simulink model "Sim17"  (R2019a)
settings: Solver=FixedStepAuto  StartTime=0.0  StopTime=10.0  FixedStep=0.0001  MaxStep=0.0001  MinStep=0.0001  RelTol=1e-3
settings Model: Creator=fbleo  LastModifiedBy=fbleo
settings SolverCC: InitialStep=0.0001

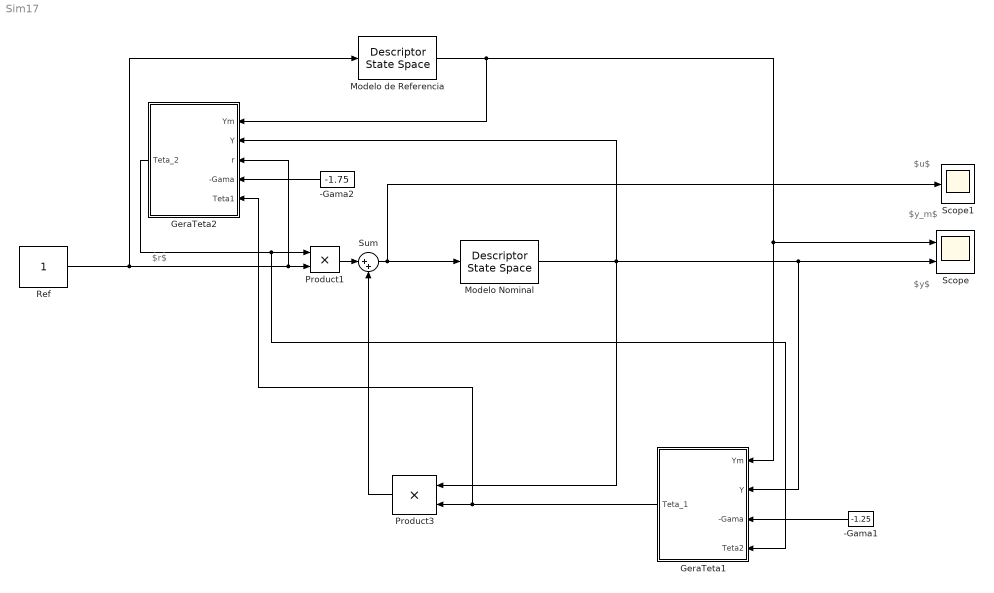
== system Sim17 ==
  note: $r$
  note: $y$
  note: $u$
  note: $y_m$
  -Gama1 : Constant  Value=-1.25
  -Gama2 : Constant  Value=-1.75
  GeraTeta1 : Subsystem
  GeraTeta2 : Subsystem
  Modelo Nominal : DescriptorStateSpace  A=-1  B=2  D=0  InitialCondition=0.5
  Modelo de Referencia : DescriptorStateSpace  A=-3  B=3  D=0  InitialCondition=0
  Product1 : Product
  Product3 : Product
  Ref : Constant
  Scope : Scope  NumInputPorts=2
  Scope1 : Scope
  Sum : Sum  Inputs=|++
  wires:
  Ref/1 -> Product1/2, GeraTeta2/3(r), Modelo de Referencia/1
  Sum/1 -> Modelo Nominal/1, Scope1/1
  GeraTeta2/1(Teta_2) -> Product1/1, GeraTeta1/4("Teta2 ")
  -Gama2/1 -> GeraTeta2/4(-Gama)
  Modelo Nominal/1 -> GeraTeta1/2(Y), Scope/2, Product3/1, GeraTeta2/2(Y)
  Product1/1 -> Sum/1
  Product3/1 -> Sum/2
  -Gama1/1 -> GeraTeta1/3(-Gama)
  Modelo de Referencia/1 -> GeraTeta1/1(Ym), Scope/1, GeraTeta2/1(Ym)
  GeraTeta1/1(Teta_1) -> GeraTeta2/5(Teta1), Product3/2

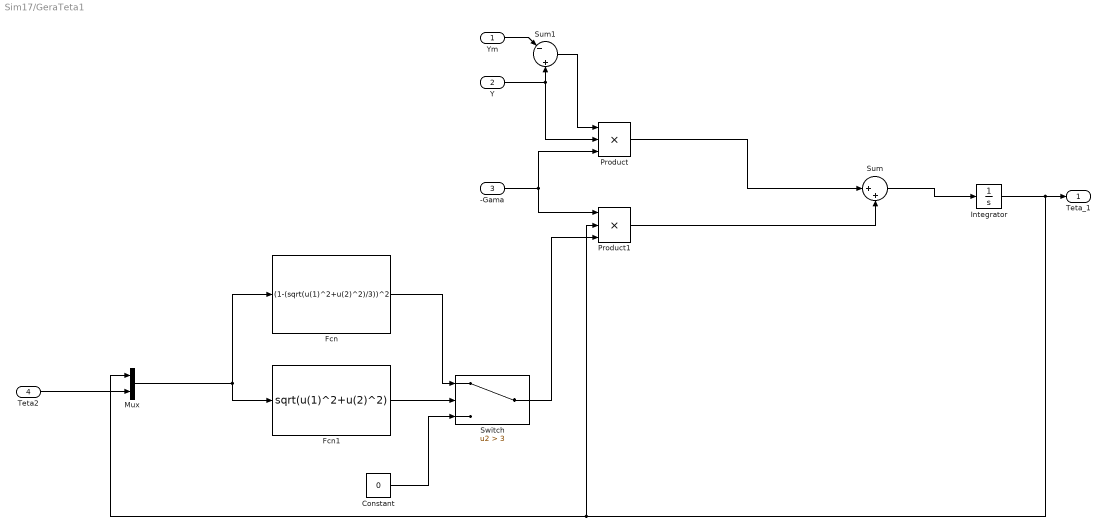
== system Sim17/GeraTeta1 ==
  Ym : Inport
  Y : Inport  Port=2
  -Gama : Inport  Port=3
  "Teta2 " : Inport  Port=4
  Constant : Constant  Value=0
  Fcn : Fcn  Expr=(1-(sqrt(u(1)^2+u(2)^2)/3))^2
  Fcn1 : Fcn  Expr=sqrt(u(1)^2+u(2)^2)
  Integrator : Integrator  InitialCondition=-0.65
  Mux : Mux  Inputs=2
  Product : Product  Inputs=3
  Product1 : Product  Inputs=3
  Sum : Sum  Inputs=|++
  Sum1 : Sum  Inputs=|-||+
  Switch : Switch  Criteria=u2 > Threshold  Threshold=3
  Teta_1 : Outport
  wires:
  Ym/1 -> Sum1/1
  Sum1/1 -> Product/1
  Y/1 -> Sum1/2, Product/2
  -Gama/1 -> Product1/1, Product/3
  Product/1 -> Sum/1
  Sum/1 -> Integrator/1
  Integrator/1 -> Mux/1, Product1/2, Teta_1/1
  "Teta2 "/1 -> Mux/2
  Switch/1 -> Product1/3
  Product1/1 -> Sum/2
  Fcn/1 -> Switch/1
  Mux/1 -> Fcn1/1, Fcn/1
  Constant/1 -> Switch/3
  Fcn1/1 -> Switch/2

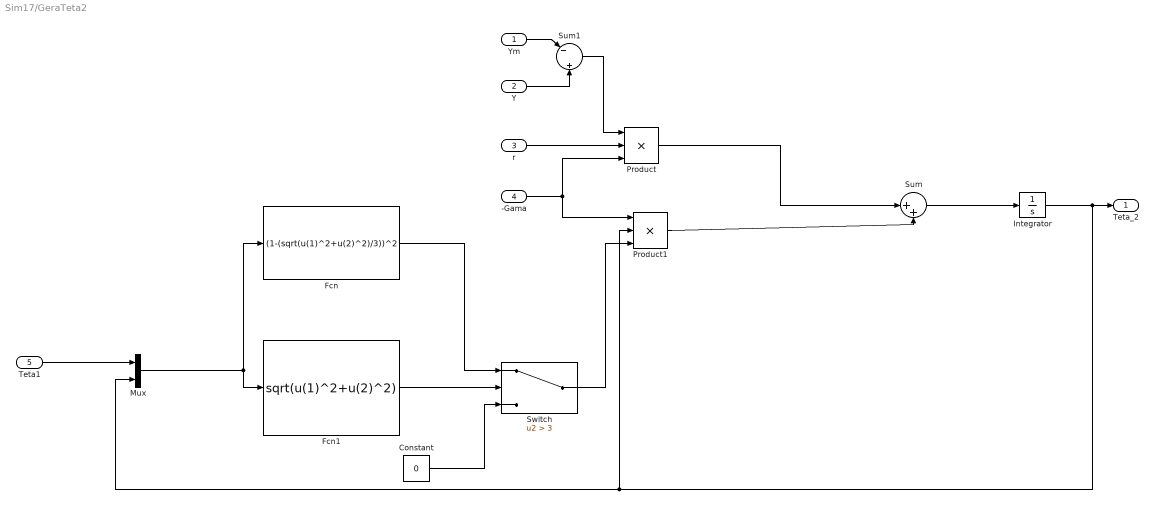
== system Sim17/GeraTeta2 ==
  Ym : Inport
  Y : Inport  Port=2
  r : Inport  Port=3
  -Gama : Inport  Port=4
  Teta1 : Inport  Port=5
  Constant : Constant  Value=0
  Fcn : Fcn  Expr=(1-(sqrt(u(1)^2+u(2)^2)/3))^2
  Fcn1 : Fcn  Expr=sqrt(u(1)^2+u(2)^2)
  Integrator : Integrator  InitialCondition=1.14
  Mux : Mux  Inputs=2
  Product : Product  Inputs=3
  Product1 : Product  Inputs=3
  Sum : Sum  Inputs=|++
  Sum1 : Sum  Inputs=|-||+
  Switch : Switch  Criteria=u2 > Threshold  Threshold=3
  Teta_2 : Outport
  wires:
  Ym/1 -> Sum1/1
  Y/1 -> Sum1/2
  Sum1/1 -> Product/1
  r/1 -> Product/2
  -Gama/1 -> Product1/1, Product/3
  Product/1 -> Sum/1
  Sum/1 -> Integrator/1
  Integrator/1 -> Mux/2, Product1/2, Teta_2/1
  Product1/1 -> Sum/2
  Mux/1 -> Fcn1/1, Fcn/1
  Fcn1/1 -> Switch/2
  Constant/1 -> Switch/3
  Switch/1 -> Product1/3
  Fcn/1 -> Switch/1
  Teta1/1 -> Mux/1
